simulink model "IBC_MPC_comment_2_5"  (R2019b)
settings: Solver=VariableStepAuto  StartTime=0.0  StopTime=0.03  RelTol=1e-3
InitFcn:
  | Load=2;
  | fs = 10e3;
  | T = 1/fs;
  | C=2600e-6;
  | L1=1000e-6;
  | L2=1000e-6*(1+normrnd(0,0.05,[1,1]));
  | L3=1000e-6*(1+normrnd(0,0.05,[1,1]));
  | alp=1-0.5;
  | V = 12;
  | L = 1000e-6;
  | D = 0.5;
  | Vg= 12;
  | R = 2;
libraries: powerlib x25, simulink x11, dspsigops x5, powerlib_meascontrol x2
settings Model: SimulationMode=accelerator  Creator=29721  LastModifiedBy=29721

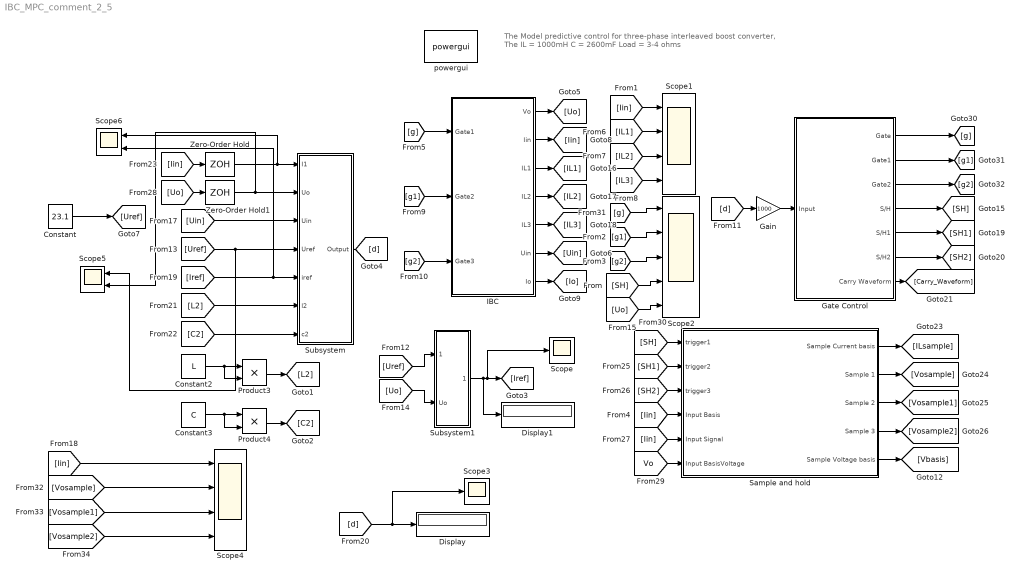
== system IBC_MPC_comment_2_5 ==
  note: The Model predictive control for three-phase interleaved boost converter,
      | The IL = 1000mH
      | C = 2600mF
      | Load = 3-4  ohms
  Constant : Constant  Value=23.1
  Constant2 : Constant  Value=L
  Constant3 : Constant  Value=C
  Display : Display
  Display1 : Display
  Gain : Gain  Gain=1000
  Gate Control : Subsystem  mask{Fs=10e3}
      mask prompts: Fs "swicthing frequency"
  IBC : Subsystem  mask{L1=L1, L2=L1, L3=L1, C=C, R=R, Vin=Vg}
  Product3 : Product
  Product4 : Product
  "Sample and hold " : Subsystem
  Scope : Scope
  Scope1 : Scope  NumInputPorts=4
  Scope2 : Scope  NumInputPorts=5
  Scope3 : Scope
  Scope4 : Scope  NumInputPorts=4
  Scope5 : Scope  NumInputPorts=2
  Scope6 : Scope  NumInputPorts=2
  Subsystem : Subsystem
  Subsystem1 : Subsystem
  Zero-Order Hold : ZeroOrderHold  SampleTime=-1
  Zero-Order Hold1 : ZeroOrderHold  SampleTime=-1
  powergui : powerlib/powergui  Priority=1  SimulationMode=Discrete  SampleTime=2.5e-8  frequency=60  Iterations=50  frequencyindice=0  Pbase=100e6  ErrMax=1e-4  UnitsV=kV  UnitsW=MW  buscounter=0  FunctionMessages=off  echomessages=off  EnableUseOfTLC=off  CurrentSourceSwitches=off  DisableSnubberDevices=off  DisableRonSwitches=off  DisableVfSwitches=off  DisplayEquations=off  AutomaticDiscreteSolvers=off  SolverType=Tustin/Backward Euler (TBE)  Interpol=off  ExternalGateDelay=off  methode=off  Ts=10  x0status=blocks  SPID=off  SwTol=0  HookPort=off  NonlinearTolerance=1e-4  nMaxIteration=100  ContinueOnMaxIteration=off  RestoreLinks=warning  ResistiveCurrentMeasurement=off  Frange=[0:2:500]  Ylog=off  Xlog=on  ShowGrid=off  save=off  variable=ZData  structure=0  ZoomFFT=off  StartTime=0.0  cycles=1  DisplayStyle=1  fundamental=60  FreqAxis=off  MaxFrequency=1000  frequencyindicesteady=1  RmsSteady=1  display=off
      settings: SourceProductName=Simscape Electrical
  wires:
  Subsystem/1(Output) -> [d]
  [Vosample2] -> Scope4/4
  "Sample and hold "/1(Sample Current basis) -> [ILsample]
  [Vosample1] -> Scope4/3
  [IL3] -> Scope1/4
  [g] -> Scope2/1
  [g1] -> IBC/2(Gate2)
  [Vosample] -> Scope4/2
  [Vo] -> "Sample and hold "/6(Input BasisVoltage)
  Constant2/1 -> Product3/2, Product3/1
  Product3/1 -> [L2]
  [g2] -> IBC/3(Gate3)
  [g] -> IBC/1(Gate1)
  [Iin] -> "Sample and hold "/4(Input Basis)
  "Sample and hold "/4(Sample 3) -> [Vosample2]
  "Sample and hold "/2(Sample 1) -> [Vosample]
  "Sample and hold "/5(Sample Voltage basis) -> [Vbasis]
  IBC/6(Uin) -> [Uin]
  [SH1] -> "Sample and hold "/2(trigger2)
  "Sample and hold "/3(Sample 2) -> [Vosample1]
  [Uin] -> Subsystem/3(Uin)
  [Iin] -> Scope4/1
  Zero-Order Hold/1 -> Scope6/1, Subsystem/1(I1)
  [SH] -> "Sample and hold "/1(trigger1)
  [Uref] -> Subsystem1/1(Uref)
  [L2] -> Subsystem/6(l2)
  IBC/7(Io) -> [Io]
  Constant/1 -> [Uref]
  [Iin] -> "Sample and hold "/5(Input Signal)
  Subsystem1/1(iref) -> Display1/1, Scope/1, [Iref]
  [Uo] -> Subsystem1/2(Uo)
  [IL2] -> Scope1/3
  IBC/3(IL1) -> [IL1]
  [IL1] -> Scope1/2
  [Iin] -> Scope1/1
  [SH2] -> "Sample and hold "/3(trigger3)
  [C2] -> Subsystem/7(c2)
  [g1] -> Scope2/2
  Product4/1 -> [C2]
  [g2] -> Scope2/3
  Zero-Order Hold1/1 -> Scope5/2, Subsystem/2(Uo)
  IBC/1(Vo) -> [Uo]
  [Uref] -> Scope5/1, Subsystem/4(Uref)
  IBC/2(Iin) -> [Iin]
  [d] -> Scope3/1, Display/1
  IBC/4(IL2) -> [IL2]
  Constant3/1 -> Product4/2, Product4/1
  IBC/5(IL3) -> [IL3]
  [SH] -> Scope2/4
  [Iref] -> Scope6/2, Subsystem/5(iref)
  [Iin] -> Zero-Order Hold/1
  [Uo] -> Zero-Order Hold1/1
  Gate Control/6(S/H2) -> [SH2]
  Gate Control/4(S/H) -> [SH]
  Gate Control/7(Carry Waveform) -> [Carry_Waveform]
  Gate Control/5(S/H1) -> [SH1]
  [d] -> Gain/1
  Gain/1 -> Gate Control/1(Input)
  Gate Control/1(Gate) -> [g]
  Gate Control/3(Gate2) -> [g2]
  Gate Control/2(Gate1) -> [g1]
  [Uo] -> Scope2/5

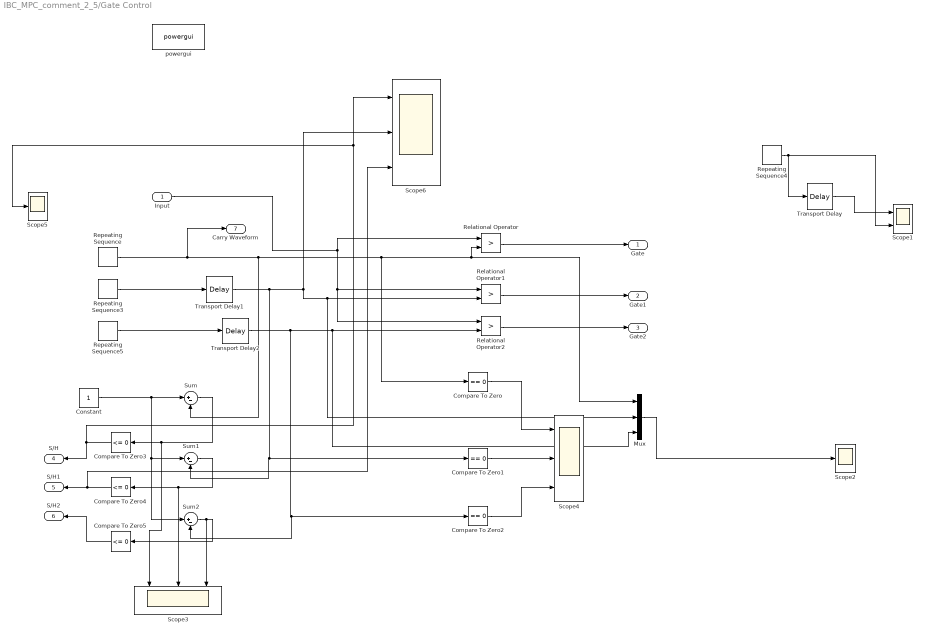
== system IBC_MPC_comment_2_5/Gate Control ==
  Input : Inport
  Compare To Zero : simulink/Logic and Bit Operations/Compare To Zero  relop===  OutDataTypeStr=boolean
  Compare To Zero1 : simulink/Logic and Bit Operations/Compare To Zero  relop===  OutDataTypeStr=boolean
  Compare To Zero2 : simulink/Logic and Bit Operations/Compare To Zero  relop===  OutDataTypeStr=boolean
  Compare To Zero3 : simulink/Logic and Bit Operations/Compare To Zero  relop=<=  OutDataTypeStr=boolean
  Compare To Zero4 : simulink/Logic and Bit Operations/Compare To Zero  relop=<=  OutDataTypeStr=boolean
  Compare To Zero5 : simulink/Logic and Bit Operations/Compare To Zero  relop=<=  OutDataTypeStr=boolean
  Constant : Constant
  Mux : Mux  Inputs=3
  Relational Operator : RelationalOperator  Operator=>  OutDataTypeStr=boolean  RndMeth=Simplest
  Relational Operator1 : RelationalOperator  Operator=>  OutDataTypeStr=boolean  RndMeth=Simplest
  Relational Operator2 : RelationalOperator  Operator=>  OutDataTypeStr=boolean  RndMeth=Simplest
  Repeating Sequence : simulink/Sources/Repeating Sequence  rep_seq_t=[0 1./Fs./2 1./Fs]  rep_seq_y=[0 1000 0]
  Repeating Sequence3 : simulink/Sources/Repeating Sequence  rep_seq_t=[1./Fs./3 5./Fs./6 4./Fs./3]  rep_seq_y=[0 1000 0]
  Repeating Sequence4 : simulink/Sources/Repeating Sequence  rep_seq_t=[0 1./100e3./2 1./100e3]  rep_seq_y=[0 1000 0]
  Repeating Sequence5 : simulink/Sources/Repeating Sequence  rep_seq_t=[2./Fs./3 7./Fs./6 5./Fs./3]  rep_seq_y=[0 1000 0]
  Scope1 : Scope  NumInputPorts=2
  Scope2 : Scope
  Scope3 : Scope  NumInputPorts=3
  Scope4 : Scope  NumInputPorts=3
  Scope5 : Scope
  Scope6 : Scope  NumInputPorts=3
  Sum : Sum  Inputs=|+-
  Sum1 : Sum  Inputs=|+-
  Sum2 : Sum  Inputs=|+-
  Transport Delay : TransportDelay  DelayTime=1./100e3./3
  Transport Delay1 : TransportDelay  DelayTime=1./Fs./3
  Transport Delay2 : TransportDelay  DelayTime=2./Fs./3
  powergui : powerlib/powergui  Priority=1  SimulationMode=Discrete  SampleTime=2.5e-8  frequency=60  Iterations=50  frequencyindice=60  Pbase=100e6  ErrMax=1e-4  UnitsV=kV  UnitsW=MW  buscounter=0  FunctionMessages=off  echomessages=off  EnableUseOfTLC=off  CurrentSourceSwitches=off  DisableSnubberDevices=off  DisableRonSwitches=off  DisableVfSwitches=off  DisplayEquations=off  AutomaticDiscreteSolvers=off  SolverType=Tustin/Backward Euler (TBE)  Interpol=off  ExternalGateDelay=off  methode=off  Ts=100  x0status=blocks  SPID=on  SwTol=0  HookPort=off  NonlinearTolerance=1e-4  nMaxIteration=100  ContinueOnMaxIteration=off  RestoreLinks=warning  ResistiveCurrentMeasurement=off  Frange=[0:2:500]  Ylog=off  Xlog=on  ShowGrid=off  save=off  variable=ZData  structure=0  ZoomFFT=off  StartTime=0.0  cycles=1  DisplayStyle=1  fundamental=60  FreqAxis=off  MaxFrequency=1000  frequencyindicesteady=1  RmsSteady=1  display=off
      settings: SourceProductName=Simscape Electrical
  Gate : Outport
  Gate1 : Outport  Port=2
  Gate2 : Outport  Port=3
  S/H : Outport  Port=4
  S/H1 : Outport  Port=5
  S/H2 : Outport  Port=6
  Carry Waveform : Outport  Port=7
  wires:
  Input/1 -> Relational Operator1/1, Relational Operator2/1, Relational Operator/1
  Compare To Zero/1 -> Scope4/1
  Relational Operator/1 -> Gate/1
  Repeating Sequence3/1 -> Transport Delay1/1
  Relational Operator1/1 -> Gate1/1
  Repeating Sequence5/1 -> Transport Delay2/1
  Repeating Sequence/1 -> Carry Waveform/1, Mux/1, Relational Operator/2, Compare To Zero/1, Sum/2
  Relational Operator2/1 -> Gate2/1
  Repeating Sequence4/1 -> Transport Delay/1, Scope1/2
  Transport Delay/1 -> Scope1/1
  Mux/1 -> Scope2/1
  Transport Delay1/1 -> Sum1/2, Compare To Zero1/1, Scope6/2, Mux/2, Relational Operator1/2
  Compare To Zero1/1 -> Scope4/2
  Compare To Zero2/1 -> Scope4/3
  Sum/1 -> Scope3/1, Compare To Zero3/1
  Sum1/1 -> Compare To Zero4/1, Scope3/2
  Transport Delay2/1 -> Sum2/2, Compare To Zero2/1, Mux/3, Relational Operator2/2
  Sum2/1 -> Scope3/3, Compare To Zero5/1
  Constant/1 -> Sum2/1, Sum1/1, Sum/1
  Compare To Zero3/1 -> Scope6/1, Scope5/1, S/H/1
  Compare To Zero4/1 -> Scope6/3, S/H1/1
  Compare To Zero5/1 -> S/H2/1

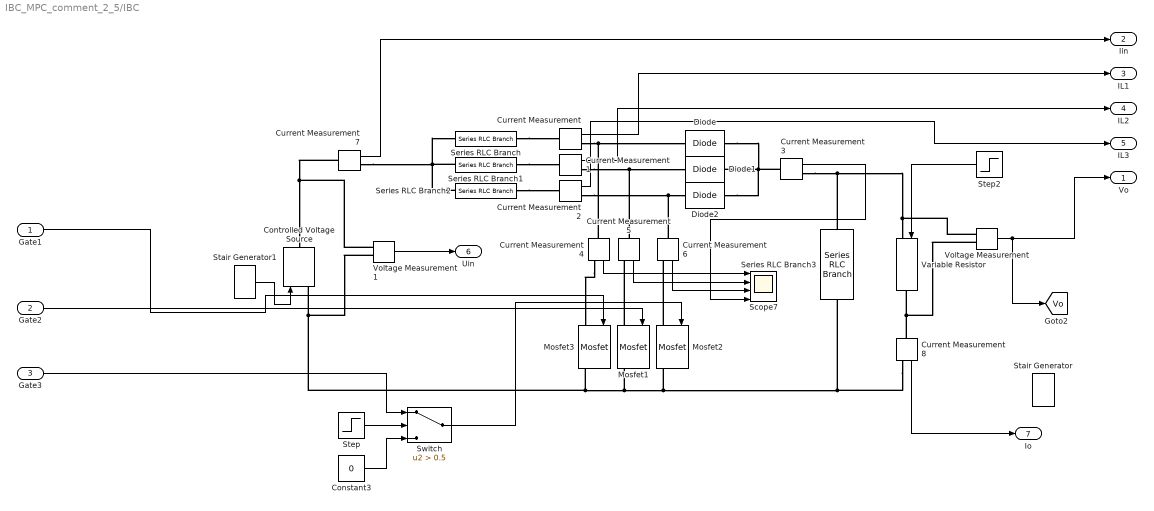
== system IBC_MPC_comment_2_5/IBC ==
  Gate1 : Inport
  Gate2 : Inport  Port=2
  Gate3 : Inport  Port=3
  Constant3 : Constant  Value=0
  Controlled Voltage Source : powerlib/Electrical Sources/Controlled Voltage Source  Initialize=on  Source_Type=AC  Amplitude=0  Phase=0  Frequency=0  Measurements=None
      settings: SourceProductName=Simscape Electrical
  Current Measurement{,1..8} (9 alike) : powerlib/Measurements/Current Measurement  PhasorSimulation=off  OutputType=Complex  PSBequivalent=0
      settings: SourceProductName=Simscape Electrical
  Diode : powerlib/Power Electronics/Diode  Ron=0.001  Lon=0  Vf=0  IC=0  UseSnubber=0  Rs=inf  Cs=250e-9  Measurements=off
      settings: SourceProductName=Simscape Electrical
  Diode1 : powerlib/Power Electronics/Diode  Ron=0.001  Lon=0  Vf=0  IC=0  UseSnubber=0  Rs=inf  Cs=250e-9  Measurements=off
      settings: SourceProductName=Simscape Electrical
  Diode2 : powerlib/Power Electronics/Diode  Ron=0.001  Lon=0  Vf=0  IC=0  UseSnubber=0  Rs=inf  Cs=250e-9  Measurements=off
      settings: SourceProductName=Simscape Electrical
  Mosfet1 : powerlib/Power Electronics/Mosfet  Ron=0.1  Lon=0  Rd=0.01  Vfd=0  IC=0  Rs=1e5  Cs=inf  Measurements=on
      settings: SourceProductName=Simscape Electrical
  Mosfet2 : powerlib/Power Electronics/Mosfet  Ron=0.1  Lon=0  Rd=0.01  Vfd=0  IC=0  Rs=1e5  Cs=inf  Measurements=on
      settings: SourceProductName=Simscape Electrical
  Mosfet3 : powerlib/Power Electronics/Mosfet  Ron=0.1  Lon=0  Rd=0.01  Vfd=0  IC=0  Rs=1e5  Cs=inf  Measurements=on
      settings: SourceProductName=Simscape Electrical
  Scope7 : Scope  NumInputPorts=4
  Series RLC Branch : powerlib/Elements/Series RLC Branch  LConnTagsString=__new0  RConnTagsString=__new0  BranchType=L  Resistance=0.14  Inductance=L1  SetiL0=off  InitialCurrent=0  Capacitance=1e-6  Setx0=off  InitialVoltage=0  Measurements=None
      settings: SourceProductName=Simscape Electrical
  Series RLC Branch1 : powerlib/Elements/Series RLC Branch  LConnTagsString=__new0  RConnTagsString=__new0  BranchType=L  Resistance=0.14  Inductance=L2  SetiL0=off  InitialCurrent=0  Capacitance=1e-6  Setx0=off  InitialVoltage=0  Measurements=None
      settings: SourceProductName=Simscape Electrical
  Series RLC Branch2 : powerlib/Elements/Series RLC Branch  LConnTagsString=__new0  RConnTagsString=__new0  BranchType=L  Resistance=0.14  Inductance=L3  SetiL0=off  InitialCurrent=0  Capacitance=1e-6  Setx0=off  InitialVoltage=0  Measurements=None
      settings: SourceProductName=Simscape Electrical
  Series RLC Branch3 : powerlib/Elements/Series RLC Branch  LConnTagsString=__new0  RConnTagsString=__new0  BranchType=C  Resistance=69e-3  Inductance=1e-3  SetiL0=off  InitialCurrent=0  Capacitance=C  Setx0=off  InitialVoltage=0  Measurements=None
      settings: SourceProductName=Simscape Electrical
  Stair Generator : powerlib_meascontrol/Pulse & Signal Generators/Stair Generator  t=[0,0.01,0.02]  e=[2,4,8]  Ts=0
      settings: SourceProductName=Simscape Electrical
  Stair Generator1 : powerlib_meascontrol/Pulse & Signal Generators/Stair Generator  t=[0,0.01,0.02]  e=[10,10,14]  Ts=0
      settings: SourceProductName=Simscape Electrical
  Step : Step  Time=0.02490  Before=1  After=0  SampleTime=0
  Step2 : Step  Time=0.2  Before=2  After=4  SampleTime=0
  Switch : Switch  Criteria=u2 > Threshold  Threshold=0.5
  Variable Resistor : powerlib/Elements/Variable Resistor  Rabsmin=1e-3
      settings: SourceProductName=Simscape Electrical  SourceProductBaseCode=PS
  Voltage Measurement : powerlib/Measurements/Voltage Measurement  PhasorSimulation=off  OutputType=Complex  PSBequivalent=0
      settings: SourceProductName=Simscape Electrical
  Voltage Measurement1 : powerlib/Measurements/Voltage Measurement  PhasorSimulation=off  OutputType=Complex  PSBequivalent=0
      settings: SourceProductName=Simscape Electrical
  Vo : Outport
  Iin : Outport  Port=2
  IL1 : Outport  Port=3
  IL2 : Outport  Port=4
  IL3 : Outport  Port=5
  Uin : Outport  Port=6
  Io : Outport  Port=7
  tag scope: Vo=global
  wires:
  Step2/1 -> Variable Resistor/1
  Current Measurement6/1 -> Scope7/3
  Current Measurement5/1 -> Scope7/2
  Current Measurement1/1 -> IL2/1
  Current Measurement4/1 -> Scope7/1
  Current Measurement2/1 -> IL3/1
  Step/1 -> Switch/2
  Switch/1 -> Mosfet2/1
  Current Measurement3/1 -> Scope7/4
  Stair Generator1/1 -> Controlled Voltage Source/1
  Gate3/1 -> Switch/1
  Voltage Measurement/1 -> [Vo], Vo/1
  Current Measurement/1 -> IL1/1
  Constant3/1 -> Switch/3
  Current Measurement7/1 -> Iin/1
  Gate1/1 -> Mosfet3/1
  Gate2/1 -> Mosfet1/1
  Voltage Measurement1/1 -> Uin/1
  Current Measurement8/1 -> Io/1
  connections:
  Series RLC Branch2/RConn1 -- Current Measurement2/LConn1
  Mosfet2/LConn1 -- Current Measurement6/RConn1
  Current Measurement7/LConn1 -- Controlled Voltage Source/RConn1 -- Voltage Measurement1/LConn1
  Series RLC Branch/RConn1 -- Current Measurement/LConn1
  Series RLC Branch1/RConn1 -- Current Measurement1/LConn1
  Mosfet1/LConn1 -- Current Measurement5/RConn1
  Current Measurement2/RConn1 -- Current Measurement6/LConn1 -- Diode2/LConn1
  Current Measurement3/RConn1 -- Series RLC Branch3/LConn1 -- Voltage Measurement/LConn1 -- Variable Resistor/LConn1
  Current Measurement4/RConn1 -- Mosfet3/LConn1
  Current Measurement7/RConn1 -- Series RLC Branch2/LConn1 -- Series RLC Branch1/LConn1 -- Series RLC Branch/LConn1
  Current Measurement1/RConn1 -- Diode1/LConn1 -- Current Measurement5/LConn1
  Current Measurement3/LConn1 -- Diode2/RConn1 -- Diode/RConn1 -- Diode1/RConn1
  Current Measurement/RConn1 -- Diode/LConn1 -- Current Measurement4/LConn1
  Mosfet3/RConn1 -- Voltage Measurement1/LConn2 -- Controlled Voltage Source/LConn1 -- Mosfet1/RConn1 -- Mosfet2/RConn1 -- Current Measurement8/RConn1 -- Series RLC Branch3/RConn1
  Voltage Measurement/LConn2 -- Variable Resistor/RConn1 -- Current Measurement8/LConn1

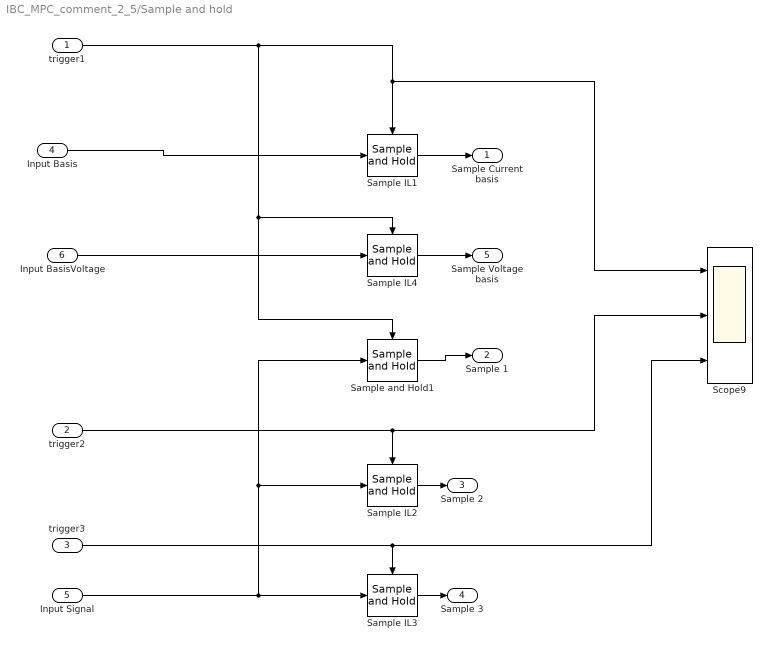
== system IBC_MPC_comment_2_5/Sample and hold  ==
  trigger1 : Inport
  trigger2 : Inport  Port=2
  trigger3 : Inport  Port=3
  Input Basis : Inport  Port=4
  Input Signal : Inport  Port=5
  Input BasisVoltage : Inport  Port=6
  Sample IL{1..4} (4 alike) : dspsigops/Sample and Hold  trig=Falling edge  initCond=0  latchinput=off
  Sample and Hold1 : dspsigops/Sample and Hold  trig=Falling edge  initCond=0  latchinput=off
  Scope9 : Scope  NumInputPorts=3
  Sample Current basis : Outport
  Sample 1 : Outport  Port=2
  Sample 2 : Outport  Port=3
  Sample 3 : Outport  Port=4
  Sample Voltage basis : Outport  Port=5
  wires:
  trigger3/1 -> Sample IL3/Trigger, Scope9/3
  Input Signal/1 -> Sample and Hold1/1, Sample IL2/1, Sample IL3/1
  Sample IL3/1 -> Sample 3/1
  trigger1/1 -> Scope9/1, Sample IL1/Trigger, Sample IL4/Trigger, Sample and Hold1/Trigger
  trigger2/1 -> Sample IL2/Trigger, Scope9/2
  Sample IL2/1 -> Sample 2/1
  Input Basis/1 -> Sample IL1/1
  Sample IL1/1 -> Sample Current basis/1
  Sample and Hold1/1 -> Sample 1/1
  Input BasisVoltage/1 -> Sample IL4/1
  Sample IL4/1 -> Sample Voltage basis/1

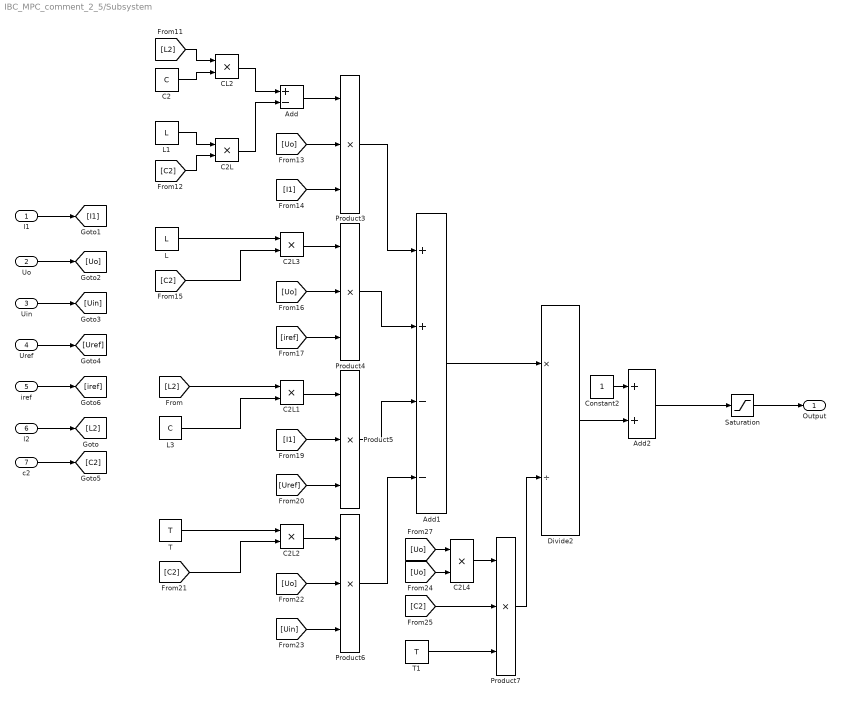
== system IBC_MPC_comment_2_5/Subsystem ==
  I1 : Inport
  Uo : Inport  Port=2
  Uin : Inport  Port=3
  Uref : Inport  Port=4
  iref : Inport  Port=5
  l2 : Inport  Port=6
  c2 : Inport  Port=7
  Add : Sum  Inputs=+-
  Add1 : Sum  Inputs=++--
  Add2 : Sum
  C2 : Constant  Value=C
  C2L{,1..4} (5 alike) : Product
  CL2 : Product
  Constant2 : Constant
  Divide2 : Product  Inputs=*/
  L : Constant  Value=L
  L1 : Constant  Value=L
  L3 : Constant  Value=C
  Product{3..7} (5 alike) : Product  Inputs=3
  Saturation : Saturate  UpperLimit=1  LowerLimit=0
  T : Constant  Value=T
  T1 : Constant  Value=T
  Output : Outport
  wires:
  C2L3/1 -> Product4/1
  [C2] -> Product7/2
  [iref] -> Product4/3
  I1/1 -> [I1]
  [L2] -> CL2/1
  L1/1 -> C2L/1
  Add/1 -> Product3/1
  Product5/1 -> Add1/3
  [C2] -> C2L3/2
  Uo/1 -> [Uo]
  [Uo] -> Product4/2
  CL2/1 -> Add/1
  Product7/1 -> Divide2/2
  Uref/1 -> [Uref]
  C2L/1 -> Add/2
  Add1/1 -> Divide2/1
  Constant2/1 -> Add2/1
  L/1 -> C2L3/1
  [I1] -> Product3/3
  [Uo] -> C2L4/1
  [L2] -> C2L1/1
  Uin/1 -> [Uin]
  iref/1 -> [iref]
  C2L2/1 -> Product6/1
  C2/1 -> CL2/2
  Product4/1 -> Add1/2
  Product3/1 -> Add1/1
  Divide2/1 -> Add2/2
  C2L1/1 -> Product5/1
  [Uo] -> Product3/2
  [Uin] -> Product6/3
  L3/1 -> C2L1/2
  [Uref] -> Product5/3
  [I1] -> Product5/2
  [C2] -> C2L2/2
  T/1 -> C2L2/1
  [Uo] -> Product6/2
  Product6/1 -> Add1/4
  C2L4/1 -> Product7/1
  [Uo] -> C2L4/2
  T1/1 -> Product7/3
  [C2] -> C2L/2
  l2/1 -> [L2]
  c2/1 -> [C2]
  Add2/1 -> Saturation/1
  Saturation/1 -> Output/1

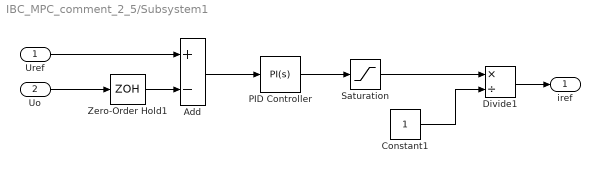
== system IBC_MPC_comment_2_5/Subsystem1 ==
  Uref : Inport
  Uo : Inport  Port=2
  Add : Sum  Inputs=+-
  Constant1 : Constant
  Divide1 : Product  Inputs=*/
  PID Controller : simulink/Continuous/PID Controller  Controller=PI  Form=Parallel  TimeDomain=Continuous-time  SampleTime=-1  IntegratorMethod=Forward Euler  FilterMethod=Forward Euler  ControllerParametersSource=internal  P=2  I=300  D=0  UseFilter=on  N=100  TunerSelectOption=Transfer Function Based (PID Tuner App)  InitialConditionSource=internal  InitialConditionForIntegrator=0  InitialConditionForFilter=0  DifferentiatorICPrevScaledInput=0  ExternalReset=none  TrackingMode=off  Kt=1  LimitOutput=off  UpperSaturationLimit=inf  LowerSaturationLimit=-inf  LinearizeAsGain=on  AntiWindupMode=none  Kb=1  POutMin=[]  POutMax=[]  IOutMin=[]  IOutMax=[]  DOutMin=[]  DOutMax=[]  NOutMin=[]  NOutMax=[]  SumOutMin=[]  SumOutMax=[]  SaturationOutMin=[]  SaturationOutMax=[]  PParamMin=[]  PParamMax=[]  IParamMin=[]  IParamMax=[]  DParamMin=[]  DParamMax=[]  NParamMin=[]  NParamMax=[]  KbParamMin=[]  KbParamMax=[]  KtParamMin=[]  KtParamMax=[]  KbOutMin=[]  KbOutMax=[]  KtOutMin=[]  KtOutMax=[]  IntegratorOutMin=[]  IntegratorOutMax=[]  FilterOutMin=[]  FilterOutMax=[]  SumI1OutMin=[]  SumI1OutMax=[]  SumI2OutMin=[]  SumI2OutMax=[]  SumI3OutMin=[]  SumI3OutMax=[]  SumI4OutMin=[]  SumI4OutMax=[]  SumDOutMin=[]  SumDOutMax=[]  DifferentiatorOutMin=[]  DifferentiatorOutMax=[]  FilterDiffOutCoefMin=[]  FilterDiffOutCoefMax=[]  ReciprocalOutMin=[]  ReciprocalOutMax=[]  SumDenOutMin=[]  SumDenOutMax=[]  SumNumOutMin=[]  SumNumOutMax=[]  DivideOutMin=[]  DivideOutMax=[]  IntegratorContinuousStateAttributes=''  IntegratorStateMustResolveToSignalObject=off  IntegratorRTWStateStorageClass=Auto  FilterContinuousStateAttributes=''  FilterStateMustResolveToSignalObject=off  FilterRTWStateStorageClass=Auto  ParallelPVariant=InternalParameters  IdealPVariant=Disabled  IVariant=InternalParameters  DVariant=Disabled  IntegratorVariant=Continuous  SatVariant=Disabled  AWVariant=Passthrough  PCopyVariant=Disabled  TRVariant=Disabled  FdbkBlocksVariant=Forward  IdealPFdbkVariant=Disabled  SatFdbkVariant=Disabled  DerivativeFilterVariant=Disabled  NVariant=Disabled  NCopyVariant=Disabled_SignalSpec  FilterICVariant=Disabled  IntegratorICVariant=InternalICs  ExternalResetVariant=Disabled  TRSumVariant=Passthrough  SumFdbkVariant=Disabled  SumVariant=Sum_PI
  Saturation : Saturate  UpperLimit=20  LowerLimit=0
  Zero-Order Hold1 : ZeroOrderHold  SampleTime=-1
  iref : Outport
  wires:
  Uo/1 -> Zero-Order Hold1/1
  Constant1/1 -> Divide1/2
  Saturation/1 -> Divide1/1
  Zero-Order Hold1/1 -> Add/2
  Divide1/1 -> iref/1
  Uref/1 -> Add/1
  Add/1 -> PID Controller/1
  PID Controller/1 -> Saturation/1
